simulink model "Nonlinear_Model"  (R2018a)
settings: Solver=VariableStepAuto  StartTime=0.0  StopTime=500  RelTol=1e-3
values from neighbouring files (symbols this model uses):
  b = 59.64    [cont_code-1.m]    (also in flight_controller.m)
  c_bar = 8.324    [cont_code-1.m]    (also in flight_controller.m)
  Clb = -0.2797    [cont_code-1.m]    (also in flight_controller.m)
  Cldelta_a = -1.368e-2    (= -0.01368)    [cont_code-1.m]    (also in flight_controller.m)
  Cldelta_r = 6.976e-3    (= 0.006976)    [cont_code-1.m]    (also in flight_controller.m)
  Clp = -0.3295    [cont_code-1.m]    (also in flight_controller.m)
  Clr = 0.3040    (= 0.304)    [cont_code-1.m]    (also in flight_controller.m)
  Cma = -1.0230    (= -1.023)    [cont_code-1.m]    (also in flight_controller.m)
  Cmdelta_e = -1.444    [cont_code-1.m]    (also in flight_controller.m)
  Cmq = -23.9200    (= -23.92)    [cont_code-1.m]    (also in flight_controller.m)
  Cmu = 0.1043    [cont_code-1.m]    (also in flight_controller.m)
  Cnb = 0.1946    [cont_code-1.m]    (also in flight_controller.m)
  Cndelta_a = -1.973e-4    (= -0.0001973)    [cont_code-1.m]    (also in flight_controller.m)
  Cndelta_r = -0.1257    [cont_code-1.m]    (also in flight_controller.m)
  Cnp = -0.04073    [cont_code-1.m]    (also in flight_controller.m)
  Cnr = -0.2737    [cont_code-1.m]    (also in flight_controller.m)
  Cwo = W / (0.5 * rho * S * Uo^2)    (= 0.654067183199)    [cont_code-1.m]    (also in flight_controller.m)
  Cxa = 0.2193    [cont_code-1.m]    (also in flight_controller.m)
  Cxdelta_e = -3.818e-6    (= -3.818e-06)    [cont_code-1.m]    (also in flight_controller.m)
  Cxdelta_p = 0.3 * Cwo    (= 0.19622015496)    [cont_code-1.m]    (also in flight_controller.m)
  Cxu = -0.1080    (= -0.108)    [cont_code-1.m]    (also in flight_controller.m)
  Cyb = -0.8771    [cont_code-1.m]    (also in flight_controller.m)
  Cydelta_r = 0.1146    [cont_code-1.m]    (also in flight_controller.m)
  Cza = -4.9200    (= -4.92)    [cont_code-1.m]    (also in flight_controller.m)
  Czdelta_e = -0.3648    [cont_code-1.m]    (also in flight_controller.m)
  Czq = -5.9210    (= -5.921)    [cont_code-1.m]    (also in flight_controller.m)
  Czu = -0.1060    (= -0.106)    [cont_code-1.m]    (also in flight_controller.m)
  g = 9.81    [cont_code-1.m]    (also in flight_controller.m)
  Ixx = 0.247e+8    (= 24700000)    [cont_code-1.m]    (also in flight_controller.m)
  Ixz = -0.212e+7    (= -2120000)    [cont_code-1.m]    (also in flight_controller.m)
  Iyy = 0.449e+8    (= 44900000)    [cont_code-1.m]    (also in flight_controller.m)
  Izz = 0.673e+8    (= 67300000)    [cont_code-1.m]    (also in flight_controller.m)
  m = W / g    (= 288660.550459)    [cont_code-1.m]    (also in flight_controller.m)
  rho = 0.3045    [cont_code-1.m]    (also in flight_controller.m)
  S = 511    [cont_code-1.m]    (also in flight_controller.m)
  Uo = 235.9    [cont_code-1.m]    (also in flight_controller.m)
libraries: simulink x2
settings Model: Creator=Navneet  LastModifiedBy=Sam
settings DebuggingCC: LibraryContextMissingDiagnostic=warning
settings SFSimCC: SimUseLocalCustomCode=on
settings RTWCC: RTWUseLocalCustomCode=on

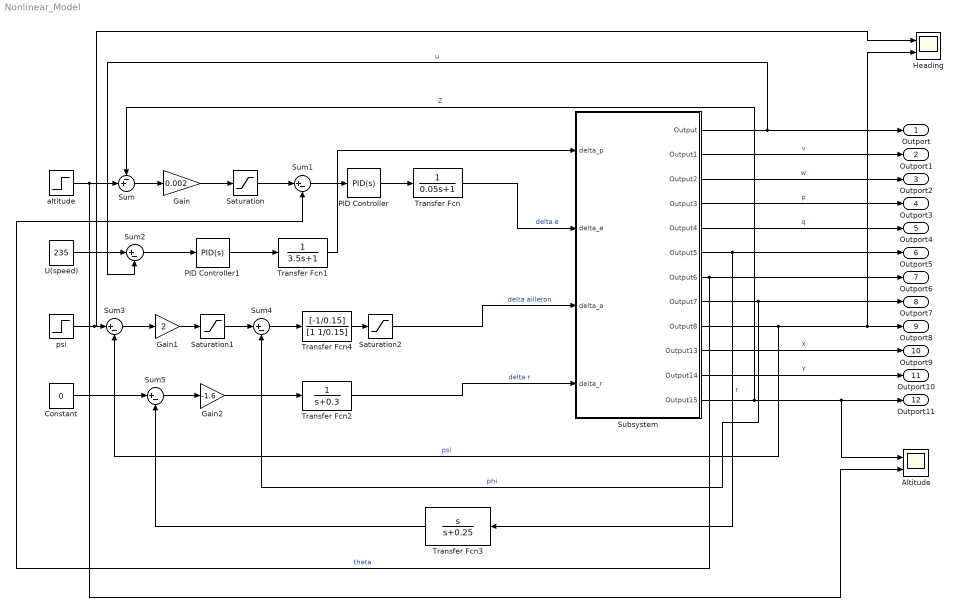
== system Nonlinear_Model ==
  Altitude : Scope  NumInputPorts=2
  Constant : Constant  Value=0
  Gain : Gain  Gain=0.002
  Gain1 : Gain  Gain=2
  Gain2 : Gain  Gain=-1.6
  Heading : Scope  NumInputPorts=2
  PID Controller : simulink/Continuous/PID Controller  Controller=PID  TimeDomain=Continuous-time  SampleTime=-1  IntegratorMethod=Forward Euler  FilterMethod=Forward Euler  Form=Parallel  UseFilter=on  ControllerParametersSource=internal  P=-84.2591740266748  I=-0.19269673269316  D=-233.839197154928  N=30.0609089938909  InitialConditionSource=internal  InitialConditionForIntegrator=0  InitialConditionForFilter=0  ExternalReset=none  LimitOutput=off  UpperSaturationLimit=inf  LowerSaturationLimit=-inf  LinearizeAsGain=on  AntiWindupMode=none  Kb=1  TrackingMode=off  Kt=1  PParamMin=[]  PParamMax=[]  IParamMin=[]  IParamMax=[]  DParamMin=[]  DParamMax=[]  NParamMin=[]  NParamMax=[]  KbParamMin=[]  KbParamMax=[]  KtParamMin=[]  KtParamMax=[]  POutMin=[]  POutMax=[]  IOutMin=[]  IOutMax=[]  DOutMin=[]  DOutMax=[]  NOutMin=[]  NOutMax=[]  KbOutMin=[]  KbOutMax=[]  KtOutMin=[]  KtOutMax=[]  IntegratorOutMin=[]  IntegratorOutMax=[]  FilterOutMin=[]  FilterOutMax=[]  SumOutMin=[]  SumOutMax=[]  SumI1OutMin=[]  SumI1OutMax=[]  SumI2OutMin=[]  SumI2OutMax=[]  SumI3OutMin=[]  SumI3OutMax=[]  SumDOutMin=[]  SumDOutMax=[]  SaturationOutMin=[]  SaturationOutMax=[]  IntegratorContinuousStateAttributes=''  IntegratorStateMustResolveToSignalObject=off  IntegratorRTWStateStorageClass=Auto  FilterContinuousStateAttributes=''  FilterStateMustResolveToSignalObject=off  FilterRTWStateStorageClass=Auto  DifferentiatorICPrevScaledInput=0  DifferentiatorOutMin=[]  DifferentiatorOutMax=[]  FilterDiffOutCoefMin=[]  FilterDiffOutCoefMax=[]  SumDenOutMin=[]  SumDenOutMax=[]  SumNumOutMin=[]  SumNumOutMax=[]  ReciprocalOutMin=[]  ReciprocalOutMax=[]  DivideOutMin=[]  DivideOutMax=[]  TunerSelectOption=Transfer Function Based (PID Tuner App)
  PID Controller1 : simulink/Continuous/PID Controller  Controller=PID  TimeDomain=Continuous-time  SampleTime=-1  IntegratorMethod=Forward Euler  FilterMethod=Forward Euler  Form=Parallel  UseFilter=on  ControllerParametersSource=internal  P=7604.02047944243  I=4742.51840690405  D=2810.70095740995  N=57.1863598290901  InitialConditionSource=internal  InitialConditionForIntegrator=0  InitialConditionForFilter=0  ExternalReset=none  LimitOutput=off  UpperSaturationLimit=inf  LowerSaturationLimit=-inf  LinearizeAsGain=on  AntiWindupMode=none  Kb=1  TrackingMode=off  Kt=1  PParamMin=[]  PParamMax=[]  IParamMin=[]  IParamMax=[]  DParamMin=[]  DParamMax=[]  NParamMin=[]  NParamMax=[]  KbParamMin=[]  KbParamMax=[]  KtParamMin=[]  KtParamMax=[]  POutMin=[]  POutMax=[]  IOutMin=[]  IOutMax=[]  DOutMin=[]  DOutMax=[]  NOutMin=[]  NOutMax=[]  KbOutMin=[]  KbOutMax=[]  KtOutMin=[]  KtOutMax=[]  IntegratorOutMin=[]  IntegratorOutMax=[]  FilterOutMin=[]  FilterOutMax=[]  SumOutMin=[]  SumOutMax=[]  SumI1OutMin=[]  SumI1OutMax=[]  SumI2OutMin=[]  SumI2OutMax=[]  SumI3OutMin=[]  SumI3OutMax=[]  SumDOutMin=[]  SumDOutMax=[]  SaturationOutMin=[]  SaturationOutMax=[]  IntegratorContinuousStateAttributes=''  IntegratorStateMustResolveToSignalObject=off  IntegratorRTWStateStorageClass=Auto  FilterContinuousStateAttributes=''  FilterStateMustResolveToSignalObject=off  FilterRTWStateStorageClass=Auto  DifferentiatorICPrevScaledInput=0  DifferentiatorOutMin=[]  DifferentiatorOutMax=[]  FilterDiffOutCoefMin=[]  FilterDiffOutCoefMax=[]  SumDenOutMin=[]  SumDenOutMax=[]  SumNumOutMin=[]  SumNumOutMax=[]  ReciprocalOutMin=[]  ReciprocalOutMax=[]  DivideOutMin=[]  DivideOutMax=[]  TunerSelectOption=Transfer Function Based (PID Tuner App)
  Saturation : Saturate  UpperLimit=3.14/18  LowerLimit=-3.14/18
  Saturation1 : Saturate  UpperLimit=3.141/6  LowerLimit=-3.141/6
  Saturation2 : Saturate
  Subsystem : Subsystem
  Sum : Sum  Inputs=-+|
  Sum{1..5} (5 alike) : Sum  Inputs=|+-
  Transfer Fcn : TransferFcn  Denominator=[0.05 1]
  Transfer Fcn1 : TransferFcn  Denominator=[3.5 1]
  Transfer Fcn2 : TransferFcn  Denominator=[1 0.3]
  Transfer Fcn3 : TransferFcn  Numerator=[1 0]  Denominator=[1 0.25]
  Transfer Fcn4 : TransferFcn  Numerator=[-1/0.15]  Denominator=[1 1/0.15]
  U(speed) : Constant  Value=235
  altitude : Step  Before=12192  After=13716  SampleTime=0
  psi : Step  After=3.14/2  SampleTime=0
  Outport : Outport
  Outport1 : Outport  Port=2
  Outport2 : Outport  Port=3
  Outport3 : Outport  Port=4
  Outport4 : Outport  Port=5
  Outport5 : Outport  Port=6
  Outport6 : Outport  Port=7
  Outport7 : Outport  Port=8
  Outport8 : Outport  Port=9
  Outport9 : Outport  Port=10
  Outport10 : Outport  Port=11
  Outport11 : Outport  Port=12
  wires:
  Subsystem/1(Output) -> Outport/1, Sum2/2  "u"
  Subsystem/2(Output1) -> Outport1/1  "v"
  Subsystem/3(Output2) -> Outport2/1  "w"
  Subsystem/4(Output3) -> Outport3/1  "p"
  Subsystem/5(Output4) -> Outport4/1  "q"
  Subsystem/6(Output5) -> Transfer Fcn3/1, Outport5/1  "r"
  Subsystem/7(Output6) -> Sum1/2, Outport6/1  "theta"
  Subsystem/8(Output7) -> Outport7/1, Sum4/2  "phi"
  Subsystem/9(Output8) -> Heading/2, Outport8/1, Sum3/2  "psi"
  Subsystem/10(Output13) -> Outport9/1  "X"
  Subsystem/11(Output14) -> Outport10/1  "Y"
  Subsystem/12(Output15) -> Sum/1, Altitude/1, Outport11/1  "Z"
  Saturation2/1 -> Subsystem/3(delta_a)  "delta ailleron"
  Transfer Fcn2/1 -> Subsystem/4(delta_r)  "delta r"
  Sum1/1 -> PID Controller/1
  PID Controller/1 -> Transfer Fcn/1
  Transfer Fcn/1 -> Subsystem/2(delta_e)  "delta e"
  Saturation/1 -> Sum1/1
  Gain/1 -> Saturation/1
  Sum/1 -> Gain/1
  altitude/1 -> Altitude/2, Sum/2
  U(speed)/1 -> Sum2/1
  Sum2/1 -> PID Controller1/1
  PID Controller1/1 -> Transfer Fcn1/1
  Transfer Fcn1/1 -> Subsystem/1(delta_p)
  Gain1/1 -> Saturation1/1
  Transfer Fcn4/1 -> Saturation2/1
  Sum4/1 -> Transfer Fcn4/1
  Saturation1/1 -> Sum4/1
  Sum3/1 -> Gain1/1
  psi/1 -> Heading/1, Sum3/1
  Sum5/1 -> Gain2/1
  Gain2/1 -> Transfer Fcn2/1
  Constant/1 -> Sum5/1
  Transfer Fcn3/1 -> Sum5/2

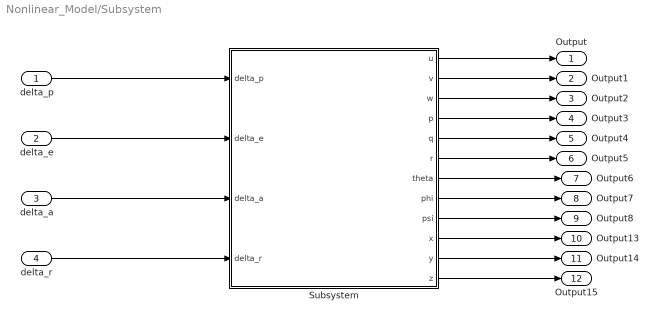
== system Nonlinear_Model/Subsystem ==
  delta_p : Inport
  delta_e : Inport  Port=2
  delta_a : Inport  Port=3
  delta_r : Inport  Port=4
  Subsystem : Subsystem
  Output : Outport
  Output1 : Outport  Port=2
  Output2 : Outport  Port=3
  Output3 : Outport  Port=4
  Output4 : Outport  Port=5
  Output5 : Outport  Port=6
  Output6 : Outport  Port=7
  Output7 : Outport  Port=8
  Output8 : Outport  Port=9
  Output13 : Outport  Port=10
  Output14 : Outport  Port=11
  Output15 : Outport  Port=12
  wires:
  Subsystem/9(psi) -> Output8/1
  delta_a/1 -> Subsystem/3(delta_a)
  Subsystem/10(x) -> Output13/1
  delta_p/1 -> Subsystem/1(delta_p)
  Subsystem/12(z) -> Output15/1
  Subsystem/11(y) -> Output14/1
  Subsystem/7(theta) -> Output6/1
  delta_r/1 -> Subsystem/4(delta_r)
  Subsystem/5(q) -> Output4/1
  Subsystem/1(u) -> Output/1
  Subsystem/4(p) -> Output3/1
  Subsystem/6(r) -> Output5/1
  Subsystem/3(w) -> Output2/1
  Subsystem/2(v) -> Output1/1
  delta_e/1 -> Subsystem/2(delta_e)
  Subsystem/8(phi) -> Output7/1

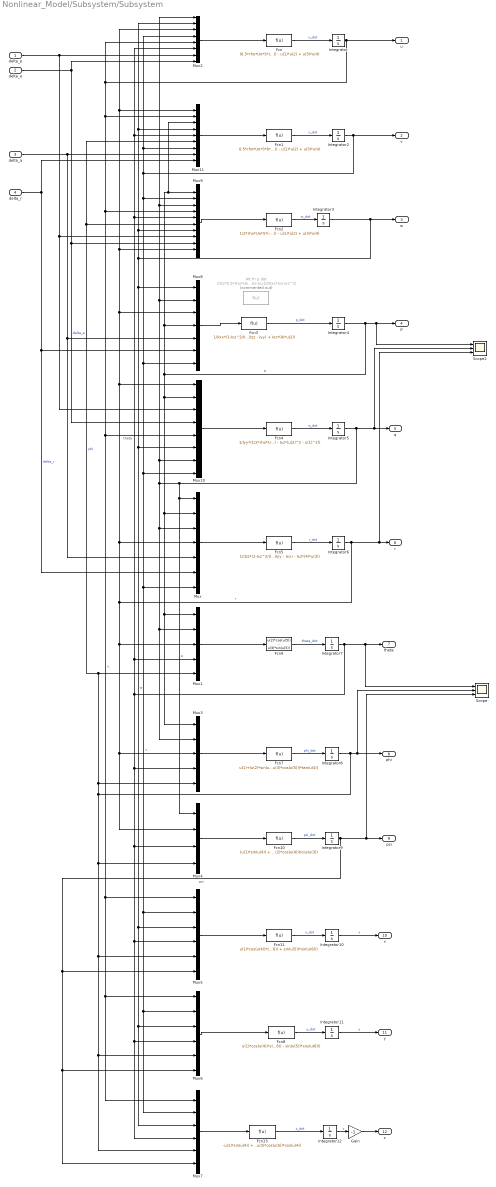
== system Nonlinear_Model/Subsystem/Subsystem ==
  delta_p : Inport
  delta_e : Inport  Port=2
  delta_a : Inport  Port=3
  delta_r : Inport  Port=4
  Alt fn p dot : Fcn  Commented=on  Expr="((Izz*0.5*rho*Uo^2*S*b*(Cldelta_a*u(5) + Cldelta_r*u(6) + Clb*u(7) + Clp*u(4) + Clr*u(3)))+(Ixz*0.5*rho*Uo^2*S*b*(Cnb*u(7) + Cndelta_a*u(5) + Cndelta_r*u(6) +Cnp*u(4) + Cnr*u(3)))  -u(2)*(Ixz*u(4)*(Iyy-Ixx-Izz)) + u(3)*(Ixz^2+Izz*(Izz-Iyy)))/(Ixx*Izz-Ixz^2)"
  Fcn : Fcn  Expr=(0.5*rho*Uo*S*(Cwo*sin(u(6))+ Cxdelta_p*u(7) + Cxdelta_e*u(8) + Cxu*u(5) - Cxa*u(2))/m) - g*sin(u(6)) - u(1)*u(2) + u(3)*u(4)
  Fcn1 : Fcn  Expr=0.5*rho*Uo*S*b*(Cydelta_r*u(9) + Cyb*u(7))/m + g*cos(u(5))*sin(u(6)) - u(1)*u(2) + u(3)*u(4)
  Fcn10 : Fcn  Expr=(u(1)*sin(u(4)) + u(2)*cos(u(4)))/cos(u(3))
  Fcn11 : Fcn  Expr=u(1)*cos(u(4))*cos(u(6)) + u(2)*(sin(u(5))*sin(u(4))*cos(u(6)) - cos(u(5))*sin(u(6))) + u(3)*(cos(u(5))*sin(u(4))*cos(u(6)) + sin(u(5))*sin(u(6)))
  Fcn13 : Fcn  Expr=-u(1)*sin(u(4)) + u(2)*sin(u(5))*cos(u(4)) + u(3)*cos(u(5))*cos(u(4))
  Fcn2 : Fcn  Expr=1/2*rho*Uo*S*(-Cwo*cos(u(5)) + Czdelta_e*u(9) + Czu*u(4) + Cza*u(7) + Czq*u(3))/m + g*cos(u(5))*cos(u(6)) - u(1)*u(2) + u(3)*u(4)
  Fcn3 : Fcn  Expr=1/(Ixx*(1-Ixz^2/(Izz*Ixx)))*(1/2*rho*Uo^2*S*b*(Cldelta_a*u(5) + Cldelta_r*u(6) + Clb*u(7) + Clp*u(4) + Clr*u(3)) + Ixz/Izz*(1/2*rho*Uo^2*S*b*(Cndelta_a*u(5) + Cndelta_r*u(6) + Cnb*u(7) + Cnp*u(4) + Cnr*u(3)) - u(2)*u(4)*(Iyy - Ixx) - Ixz*u(2)*u(3)) - u(2)*u(3)*(Izz - Iyy) + Ixz*(4)*u(2))
  Fcn4 : Fcn  Expr=1/Iyy*(1/2*rho*Uo*S*c_bar*(Cmdelta_e*u(4) + Cmu*u(5) + Cma*u(6) + Cmq*u(7)) - u(1)*u(2)*(Ixx - Izz) - Ixz*(u(2)^2 - u(1)^2))
  Fcn5 : Fcn  Expr=1/(Izz*(1-Ixz^2/(Izz*Ixx)))*(1/2*rho*Uo^2*S*b*(Cndelta_a*u(5) + Cndelta_r*u(6) + Cnb*u(7) + Cnp*u(2) + Cnr*u(4)) + Ixz/Ixx*(1/2*rho*Uo^2*S*b*(Cldelta_a*u(5) + Cldelta_r*u(6) + Clb*u(7) + Clp*u(2) + Clr*u(4)) - u(3)*u(4)*(Izz - Iyy) + Ixz*u(2)*u(3)) - u(2)*u(3)*(Iyy - Ixx) - Ixz*(4)*u(3))
  Fcn7 : Fcn  Expr=u(1)+(u(2)*sin(u(5)) + u(3)*cos(u(5)))*tan(u(4))
  Fcn8 : Fcn  Expr=u(1)*cos(u(4))*sin(u(6)) + u(2)*(sin(u(5))*sin(u(4))*sin(u(6)) + cos(u(5))*cos(u(6))) + u(3)*(cos(u(5))*sin(u(4))*sin(u(6)) - sin(u(5))*cos(u(6)))
  Fcn9 : Fcn  Expr=u(2)*cos(u(5)) - u(3)*sin(u(5))
  Gain : Gain  Gain=-1
  Integrator : Integrator  InitialCondition=235
  Integrator{2..11} (10 alike) : Integrator
  Integrator12 : Integrator  InitialCondition=-12192
  Mux : Mux  Inputs=7
  Mux1 : Mux  Inputs=5
  Mux10 : Mux  Inputs=8
  Mux11 : Mux  Inputs=9
  Mux2 : Mux  Inputs=8
  Mux3 : Mux  Inputs=5
  Mux4 : Mux
  Mux5 : Mux  Inputs=6
  Mux6 : Mux  Inputs=6
  Mux7 : Mux  Inputs=6
  Mux8 : Mux  Inputs=7
  Mux9 : Mux  Inputs=10
  Scope : Scope  NumInputPorts=3
  Scope2 : Scope  NumInputPorts=3
  u : Outport
  v : Outport  Port=2
  w : Outport  Port=3
  p : Outport  Port=4
  q : Outport  Port=5
  r : Outport  Port=6
  theta : Outport  Port=7
  phi : Outport  Port=8
  psi : Outport  Port=9
  x : Outport  Port=10
  y : Outport  Port=11
  z : Outport  Port=12
  wires:
  delta_r/1 -> Mux11/9, Mux/6, Mux8/6  "delta_r"
  delta_e/1 -> Mux2/8, Mux9/9, Mux10/4  "delta_e"
  Integrator8/1 -> Scope/2, phi/1, Mux4/4, Mux5/5, Mux6/5, Mux7/5, Mux9/6, Mux11/6, Mux1/5, Mux3/5  "phi"
  Fcn/1 -> Integrator/1  "u_dot"
  Integrator3/1 -> w/1, Mux8/1, Mux10/6, Mux5/3, Mux6/3, Mux7/3, Mux9/7, Mux11/4, Mux2/2  "w"
  Integrator6/1 -> Scope2/3, r/1, Mux4/2, Mux3/3, Mux1/3, Mux9/10, Mux11/1, Mux2/3, Mux8/3, Mux10/1, Mux/4  "r"
  Integrator10/1 -> x/1  "x"
  Integrator5/1 -> Scope2/2, q/1, Mux/3, Mux3/2, Mux1/2, Mux10/7, Mux2/1, Mux9/3, Mux8/2, Mux/1, Mux4/1  "q"
  Mux5/1 -> Fcn11/1
  Integrator9/1 -> Scope/3, psi/1, Mux5/6, Mux6/6, Mux7/6  "psi"
  Integrator/1 -> u/1, Mux5/1, Mux6/1, Mux7/1, Mux10/5, Mux9/4, Mux11/2, Mux2/5  "u"
  delta_p/1 -> Mux2/7, Mux9/8, Mux10/3
  Integrator2/1 -> v/1, Mux11/7, Mux2/4, Mux10/8, Mux5/2, Mux6/2, Mux7/2, Mux/7, Mux8/7, Mux9/2  "v"
  Fcn9/1 -> Integrator7/1  "theta_dot"
  Fcn2/1 -> Integrator3/1  "w_dot"
  Integrator4/1 -> Scope2/1, p/1, Mux8/4, Mux11/3, Mux9/1, Mux3/1, Mux1/1, Mux/2, Mux10/2  "p"
  delta_a/1 -> Mux11/8, Mux/5, Mux8/5
  Integrator7/1 -> Scope/1, theta/1, Mux2/6, Mux11/5, Mux9/5, Mux1/4, Mux4/3, Mux5/4, Mux6/4, Mux7/4, Mux3/4  "theta"
  Integrator11/1 -> y/1  "y"
  Mux11/1 -> Fcn1/1
  Mux9/1 -> Fcn2/1
  Mux4/1 -> Fcn10/1
  Fcn13/1 -> Integrator12/1  "z_dot"
  Fcn10/1 -> Integrator9/1  "psi_dot"
  Mux1/1 -> Fcn9/1
  Mux10/1 -> Fcn4/1
  Mux6/1 -> Fcn8/1
  Mux/1 -> Fcn5/1
  Fcn7/1 -> Integrator8/1  "phi_dot"
  Fcn11/1 -> Integrator10/1  "x_dot"
  Fcn4/1 -> Integrator5/1  "q_dot"
  Mux3/1 -> Fcn7/1
  Fcn1/1 -> Integrator2/1  "v_dot"
  Mux7/1 -> Fcn13/1
  Fcn5/1 -> Integrator6/1  "r_dot"
  Fcn8/1 -> Integrator11/1  "y_dot"
  Mux2/1 -> Fcn/1
  Fcn3/1 -> Integrator4/1  "p_dot"
  Mux8/1 -> Fcn3/1
  Integrator12/1 -> Gain/1  "z"
  Gain/1 -> z/1
